simulink model "RequiredWork"  (R2025b)
settings: Solver=FixedStepDiscrete  StartTime=0.0  StopTime=1  RelTol=1e-3
libraries: commrandsrc3 x8, commdigbbndpm3 x6, commchan3 x5, commsink2 x4, simulink_extras x1, dspsrcs4 x1
settings Model: Creator=sid  LastModifiedBy=sid

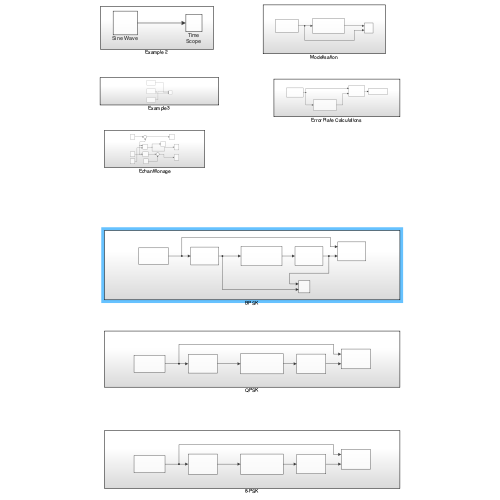
[thumbnail: Simulink's stored preview of the top-level diagram]
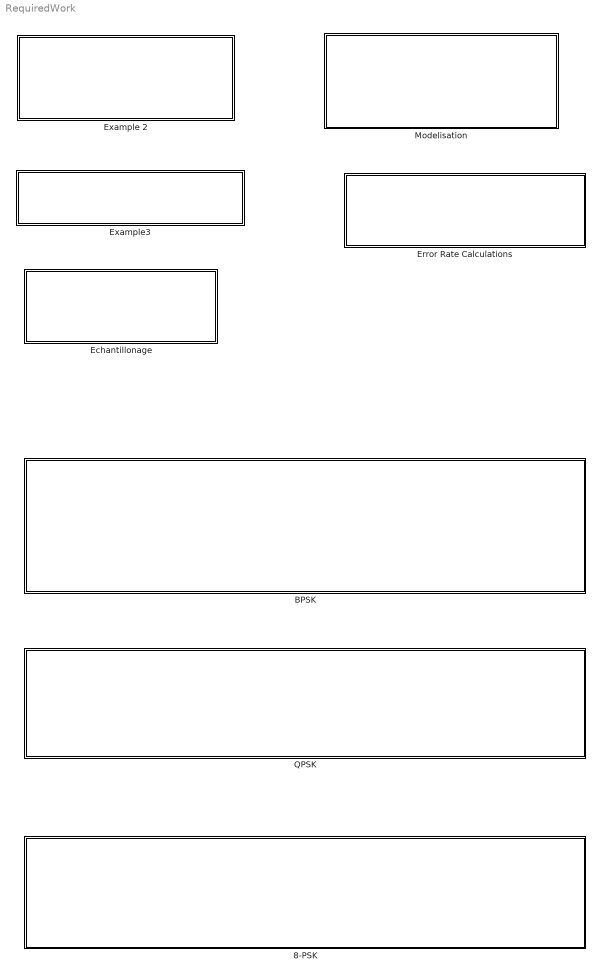
== system RequiredWork ==
  " Echantillonage" : Subsystem
  8-PSK : Subsystem
  BPSK : Subsystem
  Error Rate Calculations : Subsystem
  Example 2 : Subsystem
  Example3 : Subsystem
  Modelisation : Subsystem
  QPSK : Subsystem

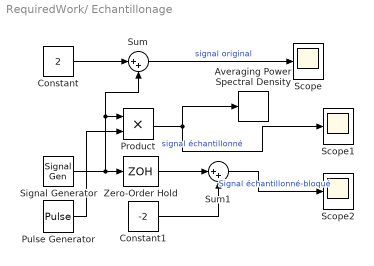
== system RequiredWork/ Echantillonage ==
  Averaging Power Spectral Density : simulink_extras/Additional Sinks/Averaging Power Spectral Density  npts=128  fftpts=512  HowOften=64  sampleT=0.0005
  Constant : Constant  Value=2
  Constant1 : Constant  Value=-2
  Product : Product
  Pulse Generator : DiscretePulseGenerator  PulseType=Time based  Period=0.001  PulseWidth=5
  Scope : Scope
      settings: ActiveDisplayYMinimum=0.75000001006390415  ActiveDisplayYMaximum=3.2499999941969149  DataLoggingVariableName=ScopeData4
  Scope1 : Scope
      settings: ActiveDisplayYMinimum=-1.2499885436627423  ActiveDisplayYMaximum=1.2499948274576453
  Scope2 : Scope
      settings: ActiveDisplayYMinimum=-3.249988543662742  ActiveDisplayYMaximum=-0.75000517254235455  DataLoggingVariableName=ScopeData5
  Signal Generator : SignalGenerator  Frequency=100  Units=rad/sec
  Sum : Sum  Inputs=|++
  Sum1 : Sum  Inputs=|++
  Zero-Order Hold : ZeroOrderHold  SampleTime=0.001
  wires:
  Constant1/1 -> Sum1/2
  Product/1 -> Scope1/1, Averaging Power Spectral Density/1  "signal échantillonné"
  Sum/1 -> Scope/1  "signal original"
  Pulse Generator/1 -> Product/2
  Zero-Order Hold/1 -> Sum1/1
  Signal Generator/1 -> Product/1, Sum/2, Zero-Order Hold/1
  Constant/1 -> Sum/1
  Sum1/1 -> Scope2/1  "Signal échantillonné-bloqué"

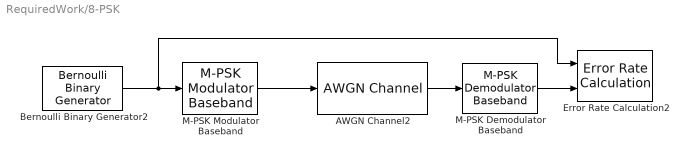
== system RequiredWork/8-PSK ==
  AWGN Channel2 : commchan3/AWGN Channel  LegacyMode=off  NoiseMethod="Signal to noise ratio  (SNR)"  noiseMode="Signal to noise ratio  (SNR)"  EbNo=10  EsNo=10  SNR=5  BitsPerSymbol=1  SignalPower=1  SpecifySymbolPeriod=off  SamplesPerSymbol=1  SymbolPeriod=1  VarianceSource=Parameter  Variance=1  RandomStream=Global stream  Seed=67  SimulateUsing=Code generation
  Bernoulli Binary Generator2 : commrandsrc3/Bernoulli Binary Generator  ProbabilityOfZero=0.5  SeedSource=Auto  Seed=0  SampleTime=0.01  SamplesPerFrame=1  OutputDataType=double  SimulateUsing=Interpreted execution
  Error Rate Calculation2 : commsink2/Error Rate Calculation  N=0  st_delay=0  cp_mode=Entire frame  subframe=[]  PMode=Workspace  WsName=mpr  RsMode2=off  stop=off  numErr=100  maxBits=1e6
      settings: LibrarySourceBlock=|
      | commhdlsink/Error Rate
      | Calculation
  M-PSK Demodulator Baseband : commdigbbndpm3/M-PSK Demodulator Baseband  M=8  OutType=Integer  DecType=Hard decision  VarSource=Dialog  Variance=1  Dec=Gray  Mapping=[0:7]  Ph=pi/8  outDtype1=Inherit via internal rule  outDtype2=Inherit via internal rule  derotateFactorWordLen=16  derotateFactorDataTypeStr=Inherit: Same word length as input  derotateFactorLastDataTypeStr=Inherit: Same word length as input
      settings: LibrarySourceBlock=|
      | commhdldigbbndpm/M-PSK
      | Demodulator
      | Baseband
  M-PSK Modulator Baseband : commdigbbndpm3/M-PSK Modulator Baseband  M=8  InType=Integer  Enc=Gray  Mapping=[0:7]  Ph=pi/8  outDtype=double  outWordLen=16  outUDDataType=sfix(16)  outFracLenMode=Best precision  outFracLen=15  outDataTypeStr=double  outLastDataTypeStr=double
      settings: LibrarySourceBlock=|
      | commhdldigbbndpm/M-PSK
      | Modulator
      | Baseband
  wires:
  M-PSK Modulator Baseband/1 -> AWGN Channel2/1
  M-PSK Demodulator Baseband/1 -> Error Rate Calculation2/2
  Bernoulli Binary Generator2/1 -> M-PSK Modulator Baseband/1, Error Rate Calculation2/1
  AWGN Channel2/1 -> M-PSK Demodulator Baseband/1

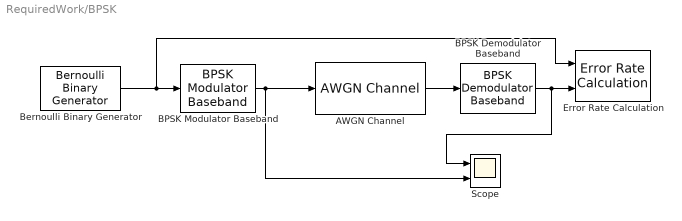
== system RequiredWork/BPSK ==
  AWGN Channel : commchan3/AWGN Channel  LegacyMode=off  NoiseMethod="Signal to noise ratio  (SNR)"  noiseMode="Signal to noise ratio  (SNR)"  EbNo=10  EsNo=10  SNR=5  BitsPerSymbol=1  SignalPower=1  SpecifySymbolPeriod=off  SamplesPerSymbol=1  SymbolPeriod=1  VarianceSource=Parameter  Variance=1  RandomStream=Global stream  Seed=67  SimulateUsing=Code generation
  BPSK Demodulator Baseband : commdigbbndpm3/BPSK Demodulator Baseband  DecType=Hard decision  VarSource=Dialog  Variance=1  Ph=0  outDtype=Inherit via internal rule  derotateFactorWordLen=16  derotateFactorDataTypeStr=Inherit: Same word length as input  derotateFactorLastDataTypeStr=Inherit: Same word length as input
      settings: LibrarySourceBlock=|
      | commhdldigbbndpm/BPSK
      | Demodulator
      | Baseband
  BPSK Modulator Baseband : commdigbbndpm3/BPSK Modulator Baseband  Ph=0  outDtype=double  outWordLen=16  outUDDataType=sfix(16)  outFracLenMode=Best precision  outFracLen=15  outDataTypeStr=double  outLastDataTypeStr=double
      settings: LibrarySourceBlock=|
      | commhdldigbbndpm/BPSK
      | Modulator
      | Baseband
  Bernoulli Binary Generator : commrandsrc3/Bernoulli Binary Generator  ProbabilityOfZero=0.5  SeedSource=Auto  Seed=0  SampleTime=0.01  SamplesPerFrame=1  OutputDataType=double  SimulateUsing=Interpreted execution
  Error Rate Calculation : commsink2/Error Rate Calculation  N=0  st_delay=0  cp_mode=Entire frame  subframe=[]  PMode=Workspace  WsName=br  RsMode2=off  stop=off  numErr=100  maxBits=1e6
      settings: LibrarySourceBlock=|
      | commhdlsink/Error Rate
      | Calculation
  Scope : Scope  NumInputPorts=2
      settings: ActiveDisplayYMinimum=-1.25  ActiveDisplayYMaximum=1.25  DataLoggingVariableName=ScopeData6
  wires:
  BPSK Modulator Baseband/1 -> Scope/2, AWGN Channel/1
  AWGN Channel/1 -> BPSK Demodulator Baseband/1
  BPSK Demodulator Baseband/1 -> Scope/1, Error Rate Calculation/2
  Bernoulli Binary Generator/1 -> Error Rate Calculation/1, BPSK Modulator Baseband/1

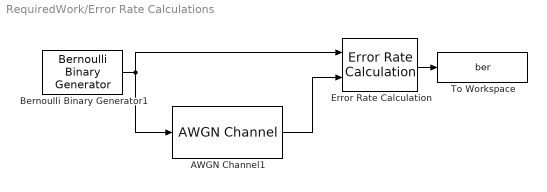
== system RequiredWork/Error Rate Calculations ==
  AWGN Channel1 : commchan3/AWGN Channel  LegacyMode=off  NoiseMethod="Signal to noise ratio  (SNR)"  noiseMode="Signal to noise ratio  (SNR)"  EbNo=10  EsNo=10  SNR=100  BitsPerSymbol=1  SignalPower=1  SpecifySymbolPeriod=off  SamplesPerSymbol=1  SymbolPeriod=1  VarianceSource=Parameter  Variance=1  RandomStream=Global stream  Seed=67  SimulateUsing=Code generation
  Bernoulli Binary Generator1 : commrandsrc3/Bernoulli Binary Generator  ProbabilityOfZero=0.5  SeedSource=Auto  Seed=0  SampleTime=0.01  SamplesPerFrame=1  OutputDataType=double  SimulateUsing=Interpreted execution
  Error Rate Calculation : commsink2/Error Rate Calculation  N=0  st_delay=0  cp_mode=Entire frame  subframe=[]  PMode=Port  WsName=BER  RsMode2=off  stop=off  numErr=100  maxBits=1e6
      settings: LibrarySourceBlock=|
      | commhdlsink/Error Rate
      | Calculation
  To Workspace : ToWorkspace  VariableName=ber  SaveFormat=Timeseries  SampleTime=-1
  wires:
  AWGN Channel1/1 -> Error Rate Calculation/2
  Bernoulli Binary Generator1/1 -> Error Rate Calculation/1, AWGN Channel1/1
  Error Rate Calculation/1 -> To Workspace/1

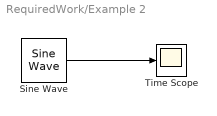
== system RequiredWork/Example 2 ==
  Sine Wave : dspsrcs4/Sine Wave  Amplitude=5  Frequency=30  Phase=0  SampleMode=Discrete  OutComplex=Real  CompMethod=Trigonometric fcn  TableSize=Speed  SampleTime=1/1000  SamplesPerFrame=100  ResetState=Restart at time zero  OutputFrames=off  dataType=double  wordLen=16  udDataType=sfix(16)  fracBitsMode=Best precision  numFracBits=15  OutDataTypeStr=double  LastOutDataTypeStr=double
  Time Scope : Scope
      settings: TimeUnits=Metric (based on Time Span)  ActiveDisplayYMinimum=-5.9441032268447271  ActiveDisplayYMaximum=5.9441032268447271  YLabel=Amplitude
  wires:
  Sine Wave/1 -> Time Scope/1

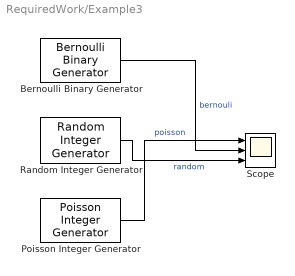
== system RequiredWork/Example3 ==
  Bernoulli Binary Generator : commrandsrc3/Bernoulli Binary Generator  ProbabilityOfZero=0.2  SeedSource=Auto  Seed=0  SampleTime=1  SamplesPerFrame=1  OutputDataType=double  SimulateUsing=Interpreted execution
  Poisson Integer Generator : commrandsrc3/Poisson Integer Generator  PoissonParameter=5  SeedSource=Auto  Seed=0  SampleTime=1  SamplesPerFrame=1  OutputDataType=double  SimulateUsing=Interpreted execution
  Random Integer Generator : commrandsrc3/Random Integer Generator  SetSize=8  SeedSource=Auto  Seed=0  SampleTime=1  SamplesPerFrame=1  OutputDataType=double  SimulateUsing=Interpreted execution
  Scope : Scope  NumInputPorts=3
      settings: ActiveDisplayYMinimum=-0.99999999999999978  ActiveDisplayYMaximum=9  DataLoggingVariableName=ScopeData2
  wires:
  Poisson Integer Generator/1 -> Scope/1  "poisson"
  Random Integer Generator/1 -> Scope/3  "random"
  Bernoulli Binary Generator/1 -> Scope/2  "bernouli"

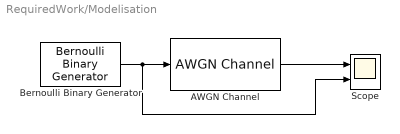
== system RequiredWork/Modelisation ==
  AWGN Channel : commchan3/AWGN Channel  LegacyMode=off  NoiseMethod="Signal to noise ratio  (SNR)"  noiseMode="Signal to noise ratio  (SNR)"  EbNo=10  EsNo=10  SNR=10  BitsPerSymbol=1  SignalPower=1  SpecifySymbolPeriod=off  SamplesPerSymbol=1  SymbolPeriod=1  VarianceSource=Parameter  Variance=1  RandomStream=Global stream  Seed=67  SimulateUsing=Code generation
  Bernoulli Binary Generator : commrandsrc3/Bernoulli Binary Generator  ProbabilityOfZero=0.5  SeedSource=Auto  Seed=0  SampleTime=0.01  SamplesPerFrame=1  OutputDataType=double  SimulateUsing=Interpreted execution
  Scope : Scope  NumInputPorts=2
      settings: ActiveDisplayYMinimum=-0.69405947084835673  ActiveDisplayYMaximum=2.0338615118997483  DataLoggingVariableName=ScopeData3
  wires:
  AWGN Channel/1 -> Scope/1
  Bernoulli Binary Generator/1 -> Scope/2, AWGN Channel/1

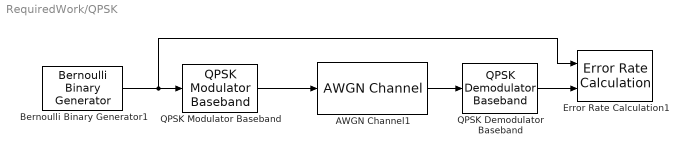
== system RequiredWork/QPSK ==
  AWGN Channel1 : commchan3/AWGN Channel  LegacyMode=off  NoiseMethod="Signal to noise ratio  (SNR)"  noiseMode="Signal to noise ratio  (SNR)"  EbNo=10  EsNo=10  SNR=5  BitsPerSymbol=1  SignalPower=1  SpecifySymbolPeriod=off  SamplesPerSymbol=1  SymbolPeriod=1  VarianceSource=Parameter  Variance=1  RandomStream=Global stream  Seed=67  SimulateUsing=Code generation
  Bernoulli Binary Generator1 : commrandsrc3/Bernoulli Binary Generator  ProbabilityOfZero=0.5  SeedSource=Auto  Seed=0  SampleTime=0.01  SamplesPerFrame=1  OutputDataType=double  SimulateUsing=Interpreted execution
  Error Rate Calculation1 : commsink2/Error Rate Calculation  N=0  st_delay=0  cp_mode=Entire frame  subframe=[]  PMode=Workspace  WsName=qr  RsMode2=off  stop=off  numErr=100  maxBits=1e6
      settings: LibrarySourceBlock=|
      | commhdlsink/Error Rate
      | Calculation
  QPSK Demodulator Baseband : commdigbbndpm3/QPSK Demodulator Baseband  OutType=Integer  DecType=Hard decision  VarSource=Dialog  Variance=1  Dec=Gray  Ph=pi/4  outDtype1=Inherit via internal rule  outDtype2=Inherit via internal rule  derotateFactorWordLen=16  derotateFactorDataTypeStr=Inherit: Same word length as input  derotateFactorLastDataTypeStr=Inherit: Same word length as input
      settings: LibrarySourceBlock=|
      | commhdldigbbndpm/QPSK
      | Demodulator
      | Baseband
  QPSK Modulator Baseband : commdigbbndpm3/QPSK Modulator Baseband  InType=Integer  Enc=Gray  Ph=pi/4  outDtype=double  outWordLen=16  outUDDataType=sfix(16)  outFracLenMode=Best precision  outFracLen=15  outDataTypeStr=double  outLastDataTypeStr=double
      settings: LibrarySourceBlock=|
      | commhdldigbbndpm/QPSK
      | Modulator
      | Baseband
  wires:
  Bernoulli Binary Generator1/1 -> QPSK Modulator Baseband/1, Error Rate Calculation1/1
  AWGN Channel1/1 -> QPSK Demodulator Baseband/1
  QPSK Modulator Baseband/1 -> AWGN Channel1/1
  QPSK Demodulator Baseband/1 -> Error Rate Calculation1/2
